simulink model "LBR_MED_CLIK_Simul"  (R2026a)
settings: Solver=VariableStepAuto
settings Model: Creator=ivovilamowski  LastModifiedBy=ivovilamowski

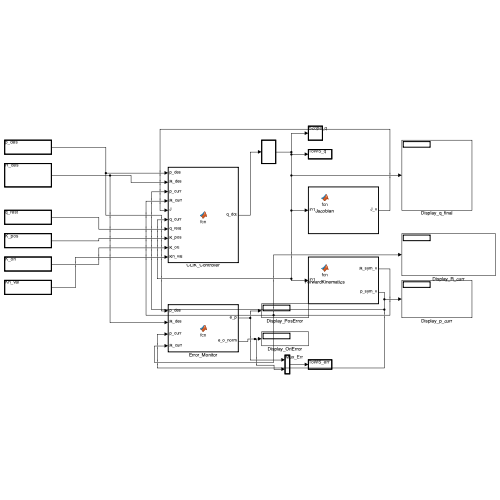
[thumbnail: Simulink's stored preview of the top-level diagram]
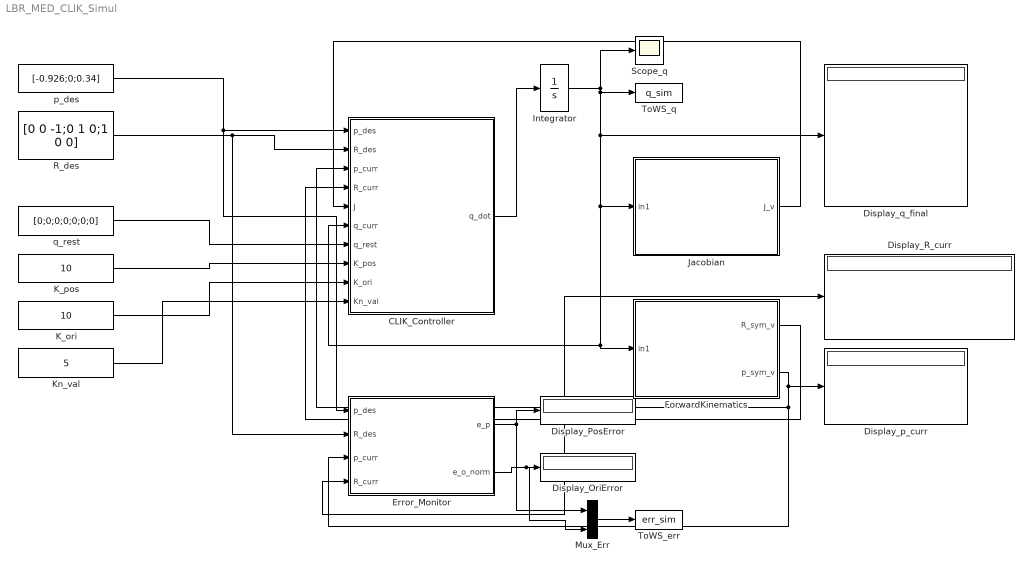
== system LBR_MED_CLIK_Simul ==
  CLIK_Controller : MATLAB Function  TreatAsAtomicUnit=on
  Display_OriError : Display
  Display_PosError : Display
  Display_R_curr : Display
  Display_p_curr : Display
  Display_q_final : Display
  Error_Monitor : MATLAB Function  TreatAsAtomicUnit=on
  ForwardKinematics : MATLAB Function  TreatAsAtomicUnit=on
  Integrator : Integrator  InitialCondition=[0;0.2;0;-0.2;0;0.2;0]
  Jacobian : MATLAB Function  TreatAsAtomicUnit=on
  K_ori : Constant  Value=10
  K_pos : Constant  Value=10
  Kn_val : Constant  Value=5
  Mux_Err : Mux  Inputs=2
  R_des : Constant  Value=[0 0 -1;0 1 0;1 0 0]
  Scope_q : Scope
  ToWS_err : ToWorkspace  VariableName=err_sim  SaveFormat=Timeseries  SampleTime=-1
  ToWS_q : ToWorkspace  VariableName=q_sim  SaveFormat=Timeseries  SampleTime=-1
  p_des : Constant  Value=[-0.926;0;0.34]
  q_rest : Constant  Value=[0;0;0;0;0;0;0]
  wires:
  Integrator/1 -> ToWS_q/1, CLIK_Controller/6(q_curr), ForwardKinematics/1(in1), Jacobian/1(in1), Display_q_final/1, Scope_q/1
  ForwardKinematics/1(R_sym_v) -> Error_Monitor/4(R_curr), Display_R_curr/1, CLIK_Controller/4(R_curr)
  ForwardKinematics/2(p_sym_v) -> Error_Monitor/3(p_curr), CLIK_Controller/3(p_curr), Display_p_curr/1
  Jacobian/1(J_v) -> CLIK_Controller/5(J)
  CLIK_Controller/1(q_dot) -> Integrator/1
  p_des/1 -> Error_Monitor/1(p_des), CLIK_Controller/1(p_des)
  R_des/1 -> Error_Monitor/2(R_des), CLIK_Controller/2(R_des)
  q_rest/1 -> CLIK_Controller/7(q_rest)
  K_pos/1 -> CLIK_Controller/8(K_pos)
  K_ori/1 -> CLIK_Controller/9(K_ori)
  Kn_val/1 -> CLIK_Controller/10(Kn_val)
  Error_Monitor/1(e_p) -> Display_PosError/1, Mux_Err/1
  Error_Monitor/2(e_o_norm) -> Mux_Err/2, Display_OriError/1
  Mux_Err/1 -> ToWS_err/1

== matlab function LBR_MED_CLIK_Simul/ForwardKinematics ==
  data: in1 input; R_sym_v output; p_sym_v output
function [R_sym_v,p_sym_v] = ForwardKinematics(in1)
%#codegen

%    This function was generated by the Symbolic Math Toolbox version 26.1.
%    04-Jun-2026 17:34:25

% in1 = complex(in1);  % if required to enforce complex operations
q1 = in1(1,:);
q2 = in1(2,:);
q3 = in1(3,:);
q4 = in1(4,:);
q5 = in1(5,:);
q6 = in1(6,:);
q7 = in1(7,:);
t2 = cos(q1);
t3 = cos(q2);
t4 = cos(q3);
t5 = cos(q4);
t6 = cos(q5);
t7 = cos(q6);
t8 = cos(q7);
t9 = sin(q1);
t10 = sin(q2);
t11 = sin(q3);
t12 = sin(q4);
t13 = sin(q5);
t14 = sin(q6);
t15 = sin(q7);
t16 = t2.*t4;
t17 = t3.*t5;
t18 = t2.*t11;
t19 = t4.*t9;
t20 = t3.*t12;
t21 = t9.*t11;
t22 = t9.*t10.*t12;
t23 = t10.*t11.*t13;
t27 = t2.*t5.*t10;
t28 = t4.*t5.*t10;
t30 = t2.*t10.*t12;
t31 = t5.*t9.*t10;
t32 = t4.*t10.*t12;
t33 = t6.*t10.*t11;
t24 = t3.*t16;
t25 = t3.*t18;
t26 = t3.*t19;
t29 = t3.*t21;
t35 = -t28;
t42 = t17+t32;
t34 = -t24;
t36 = -t29;
t40 = t18+t26;
t41 = t19+t25;
t45 = t20+t35;
t50 = t14.*t42;
t43 = t16+t36;
t44 = t21+t34;
t46 = t5.*t40;
t47 = t6.*t41;
t48 = t12.*t40;
t49 = t13.*t41;
t54 = t6.*t45;
t57 = t13.*t45;
t51 = t5.*t44;
t52 = t6.*t43;
t55 = t12.*t44;
t56 = t13.*t43;
t60 = t22+t46;
t62 = t23+t54;
t70 = -t14.*(t31-t48);
t63 = t27+t55;
t64 = t6.*t60;
t65 = t13.*t60;
t69 = t7.*t62;
t71 = -t6.*(t30-t51);
t68 = t14.*t63;
t73 = t56+t64;
t74 = t49+t71;
t77 = t7.*t73;
t79 = t7.*t74;
t80 = t70+t77;
t81 = t68+t79;
R_sym_v = reshape([-t15.*(t47+t13.*(t30-t51))-t8.*t81,t8.*t80+t15.*(t52-t65),-t15.*(t33-t57)+t8.*(t50-t69),-t8.*(t47+t13.*(t30-t51))+t15.*t81,-t15.*t80+t8.*(t52-t65),-t8.*(t33-t57)-t15.*(t50-t69),-t7.*t63+t14.*t74,-t14.*t73-t7.*(t31-t48),t7.*t42+t14.*t62],[3,3]);
if nargout > 1
    p_sym_v = [t27.*(-2.0./5.0)-t55.*(2.0./5.0)-t2.*t10.*(2.0./5.0)-t7.*t63.*(6.3e+1./5.0e+2)+t14.*t74.*(6.3e+1./5.0e+2);t31.*(-2.0./5.0)+t48.*(2.0./5.0)-t9.*t10.*(2.0./5.0)-t14.*t73.*(6.3e+1./5.0e+2)-t7.*(t31-t48).*(6.3e+1./5.0e+2);t3.*(2.0./5.0)+t17.*(2.0./5.0)+t32.*(2.0./5.0)+t7.*t42.*(6.3e+1./5.0e+2)+t14.*t62.*(6.3e+1./5.0e+2)+1.7e+1./5.0e+1];
end
end

== matlab function LBR_MED_CLIK_Simul/CLIK_Controller ==
  data: p_des input size=[3, 1]; q_dot output size=[7, 1]; R_des input size=[3, 3]; p_curr input size=[3, 1]; R_curr input size=[3, 3]; J input size=[6, 7]; q_curr input size=[7, 1]; q_rest input size=[7, 1]; K_pos input size=1; K_ori input size=1; Kn_val input size=1
function q_dot = clik_controller(p_des, R_des, p_curr, R_curr, J, q_curr, q_rest, K_pos, K_ori, Kn_val)
    q_dot = clik_controller_logic(p_des, R_des, p_curr, R_curr, J, q_curr, q_rest, K_pos, K_ori, Kn_val);
end

== matlab function LBR_MED_CLIK_Simul/Jacobian ==
  data: in1 input; J_v output
function J_v = Jacobian(in1)
%#codegen

%    This function was generated by the Symbolic Math Toolbox version 26.1.
%    04-Jun-2026 17:34:26

% in1 = complex(in1);  % if required to enforce complex operations
q1 = in1(1,:);
q2 = in1(2,:);
q3 = in1(3,:);
q4 = in1(4,:);
q5 = in1(5,:);
q6 = in1(6,:);
t2 = cos(q1);
t3 = cos(q2);
t4 = cos(q3);
t5 = cos(q4);
t6 = cos(q5);
t7 = cos(q6);
t8 = sin(q1);
t9 = sin(q2);
t10 = sin(q3);
t11 = sin(q4);
t12 = sin(q5);
t13 = sin(q6);
t14 = t2.*t4;
t15 = t3.*t5;
t16 = t2.*t10;
t17 = t4.*t8;
t18 = t3.*t11;
t19 = t8.*t10;
t20 = t3.*(2.0./5.0);
t21 = t8.*t9.*t11;
t22 = t9.*t10.*t12;
t26 = t2.*t5.*t9;
t27 = t4.*t5.*t9;
t29 = t2.*t9.*t11;
t30 = t5.*t8.*t9;
t31 = t4.*t9.*t11;
t32 = t6.*t9.*t10;
t23 = t3.*t14;
t24 = t3.*t16;
t25 = t3.*t17;
t28 = t3.*t19;
t33 = t15.*(2.0./5.0);
t35 = -t27;
t38 = -t30;
t40 = t26.*(2.0./5.0);
t41 = t30.*(2.0./5.0);
t42 = t31.*(2.0./5.0);
t45 = t15+t31;
t34 = -t23;
t36 = -t28;
t43 = t16+t25;
t44 = t17+t24;
t48 = t18+t35;
t62 = t7.*t45.*(6.3e+1./5.0e+2);
t46 = t14+t36;
t47 = t19+t34;
t49 = t5.*t43;
t50 = t6.*t44;
t51 = t11.*t43;
t52 = t12.*t44;
t55 = t6.*t48;
t58 = t12.*t48;
t53 = t5.*t47;
t54 = t6.*t46;
t56 = t11.*t47;
t57 = t12.*t46;
t59 = t51.*(2.0./5.0);
t63 = t21+t49;
t64 = t38+t51;
t65 = t22+t55;
t60 = -t54;
t61 = t56.*(2.0./5.0);
t66 = t26+t56;
t67 = t6.*t63;
t68 = t12.*t63;
t71 = -t6.*(t29-t53);
t75 = t13.*t65.*(6.3e+1./5.0e+2);
t73 = t7.*t66.*(6.3e+1./5.0e+2);
t76 = t57+t67;
t77 = t52+t71;
t78 = t60+t68;
t82 = t62+t75;
t79 = t13.*t76.*(6.3e+1./5.0e+2);
t81 = t13.*t77.*(6.3e+1./5.0e+2);
t84 = t33+t42+t82;
t83 = -t81;
t85 = t20+t84;
mt1 = [t41-t59+t79+t8.*t9.*(2.0./5.0)+t7.*(t30-t51).*(6.3e+1./5.0e+2),-t40-t61-t73+t81-t2.*t9.*(2.0./5.0),0.0,0.0,0.0,1.0,-t2.*t85,-t8.*t85,t9.*(-2.0./5.0)-t5.*t9.*(2.0./5.0)+t4.*t18.*(2.0./5.0)-t5.*t7.*t9.*(6.3e+1./5.0e+2)+t4.*t7.*t18.*(6.3e+1./5.0e+2)+t3.*t10.*t12.*t13.*(6.3e+1./5.0e+2)-t4.*t6.*t13.*t15.*(6.3e+1./5.0e+2)-t6.*t9.*t11.*t13.*(6.3e+1./5.0e+2),t8,-t2,0.0];
mt2 = [t11.*t17.*(-2.0./5.0)-t16.*t18.*(2.0./5.0)-t7.*t11.*t17.*(6.3e+1./5.0e+2)-t7.*t16.*t18.*(6.3e+1./5.0e+2)-t12.*t13.*t19.*(6.3e+1./5.0e+2)+t12.*t13.*t23.*(6.3e+1./5.0e+2)+t5.*t6.*t13.*t17.*(6.3e+1./5.0e+2)+t6.*t13.*t15.*t16.*(6.3e+1./5.0e+2),t11.*t14.*(2.0./5.0)-t18.*t19.*(2.0./5.0)+t7.*t11.*t14.*(6.3e+1./5.0e+2)+t12.*t13.*t16.*(6.3e+1./5.0e+2)-t7.*t18.*t19.*(6.3e+1./5.0e+2)+t12.*t13.*t25.*(6.3e+1./5.0e+2)-t5.*t6.*t13.*t14.*(6.3e+1./5.0e+2)+t6.*t13.*t15.*t19.*(6.3e+1./5.0e+2),t9.*(t10.*t11.*2.0e+2+t7.*t10.*t11.*6.3e+1-t4.*t12.*t13.*6.3e+1-t5.*t6.*t10.*t13.*6.3e+1).*(-1.0./5.0e+2),-t2.*t9];
mt3 = [-t8.*t9,t3,t46.*t84-t9.*t10.*(t41-t59+t79+t7.*(t30-t51).*(6.3e+1./5.0e+2)),t44.*t84+t9.*t10.*(t40+t61+t73+t83),t18.*(-2.0./5.0)+t27.*(2.0./5.0)-t7.*t18.*(6.3e+1./5.0e+2)+t7.*t27.*(6.3e+1./5.0e+2)+t6.*t13.*t15.*(6.3e+1./5.0e+2)+t6.*t13.*t31.*(6.3e+1./5.0e+2),-t44,t46,-t9.*t10,t13.*(t6.*t17+t6.*t24+t12.*t29-t5.*t12.*t19+t12.*t14.*t15).*(6.3e+1./5.0e+2),t13.*(-t6.*t14+t12.*t21+t6.*t28+t5.*t12.*t16+t12.*t15.*t17).*(6.3e+1./5.0e+2),t13.*(t32-t12.*t18+t12.*t27).*(6.3e+1./5.0e+2),-t66,t64,t45];
mt4 = [(t79+t7.*(t30-t51).*(6.3e+1./5.0e+2)).*(t32-t58)-t82.*(t54-t68),-t82.*(t50+t12.*(t29-t53))-(t73+t83).*(t32-t58),t13.*t15.*(-6.3e+1./5.0e+2)+t7.*t22.*(6.3e+1./5.0e+2)-t13.*t31.*(6.3e+1./5.0e+2)+t6.*t7.*t18.*(6.3e+1./5.0e+2)-t6.*t7.*t27.*(6.3e+1./5.0e+2),t50+t12.*(t29-t53),t78,t32-t58,0.0,0.0,0.0,-t7.*t66+t13.*t77,-t13.*t76-t7.*(t30-t51),t7.*t45+t13.*t65];
J_v = reshape([mt1,mt2,mt3,mt4],6,7);
end

== matlab function LBR_MED_CLIK_Simul/Error_Monitor ==
  data: p_des input; e_p output; R_des input; p_curr input; R_curr input; e_o_norm output
function [e_p, e_o_norm] = error_calc(p_des, R_des, p_curr, R_curr)
    e_p = norm(p_des - p_curr);
    n_e = R_curr(:,1); s_e = R_curr(:,2); a_e = R_curr(:,3);
    n_d = R_des(:,1); s_d = R_des(:,2); a_d = R_des(:,3);
    e_o = 0.5 * (cross(n_e, n_d) + cross(s_e, s_d) + cross(a_e, a_d));
    e_o_norm = norm(e_o);
end
